simulink model "Robot_diferencial"  (R2017b)
settings: Solver=VariableStepAuto  StartTime=0.0  StopTime=Tsim  MaxStep=1e-2  MinStep=1e-5  RelTol=1e-3
values from neighbouring files (symbols this model uses):
  CI = [0 0 0]    [graf.m]
settings Model: Creator=Raúl  LastModifiedBy=Raúl

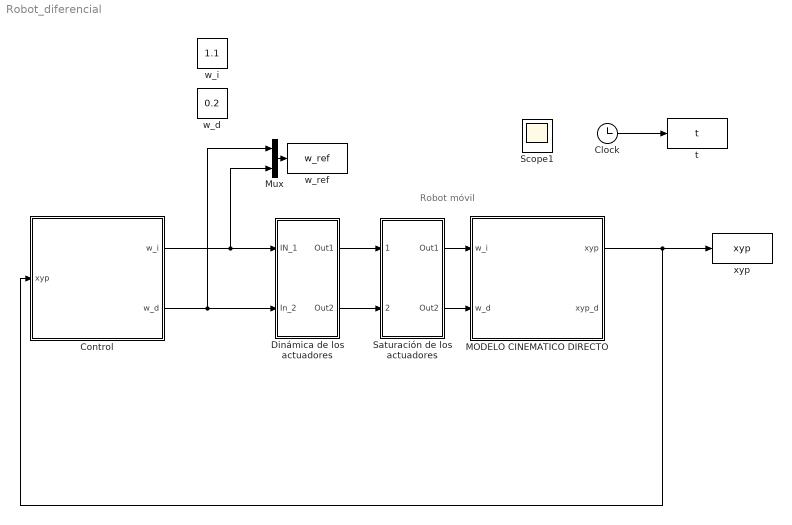
== system Robot_diferencial ==
  note: Robot móvil
  Clock : Clock
  "Control " : Subsystem
  Dinámica de los actuadores : Subsystem
  MODELO CINEMATICO DIRECTO : Subsystem
  Mux : Mux  Inputs=2
  Saturación de los actuadores : Subsystem
  Scope1 : Scope  NumInputPorts=2
  t : ToWorkspace  VariableName=t  SampleTime=-1
  w_d : Constant  Value=0.2
  w_i : Constant  Value=1.1
  w_ref : ToWorkspace  VariableName=w_ref  SampleTime=-1
  xyp : ToWorkspace  VariableName=xyp  SampleTime=-1
  wires:
  MODELO CINEMATICO DIRECTO/1(xyp) -> "Control "/1(xyp), xyp/1
  Clock/1 -> t/1
  Saturación de los actuadores/1(Out1) -> MODELO CINEMATICO DIRECTO/1(w_i)
  Saturación de los actuadores/2(Out2) -> MODELO CINEMATICO DIRECTO/2(w_d)
  Dinámica de los actuadores/1(Out1) -> Saturación de los actuadores/1(w_i_ref)
  Dinámica de los actuadores/2(Out2) -> Saturación de los actuadores/2(w_d_ref)
  "Control "/1(w_i) -> Mux/2, Dinámica de los actuadores/1(IN_1)
  "Control "/2(w_d) -> Mux/1, Dinámica de los actuadores/2(In_2)
  Mux/1 -> w_ref/1

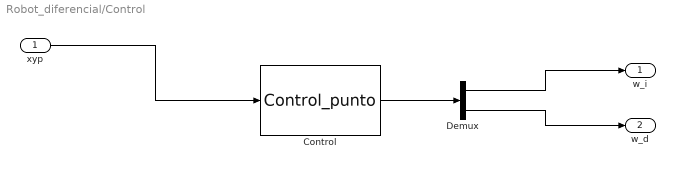
== system Robot_diferencial/Control  ==
  xyp : Inport
  "Control " : MATLABFcn  MATLABFcn=Control_punto
  Demux : Demux  Outputs=2
  w_i : Outport
  w_d : Outport  Port=2
  wires:
  Demux/1 -> w_i/1
  Demux/2 -> w_d/1
  "Control "/1 -> Demux/1
  xyp/1 -> "Control "/1

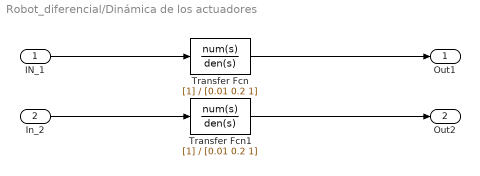
== system Robot_diferencial/Dinámica de los actuadores ==
  IN_1 : Inport
  In_2 : Inport  Port=2
  Transfer Fcn : TransferFcn  Denominator=[0.01 0.2 1]
  Transfer Fcn1 : TransferFcn  Denominator=[0.01 0.2 1]
  Out1 : Outport
  Out2 : Outport  Port=2
  wires:
  Transfer Fcn1/1 -> Out2/1
  In_2/1 -> Transfer Fcn1/1
  Transfer Fcn/1 -> Out1/1
  IN_1/1 -> Transfer Fcn/1

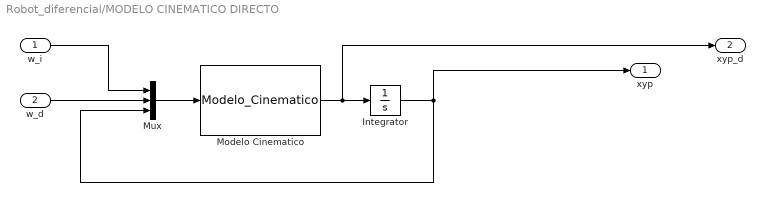
== system Robot_diferencial/MODELO CINEMATICO DIRECTO ==
  w_i : Inport
  w_d : Inport  Port=2
  Integrator : Integrator  InitialCondition=CI
  "Modelo Cinematico " : MATLABFcn  MATLABFcn=Modelo_Cinematico
  Mux : Mux  Inputs=3
  xyp : Outport
  xyp_d : Outport  Port=2
  wires:
  "Modelo Cinematico "/1 -> xyp_d/1, Integrator/1
  w_i/1 -> Mux/1
  Integrator/1 -> xyp/1, Mux/3
  Mux/1 -> "Modelo Cinematico "/1
  w_d/1 -> Mux/2

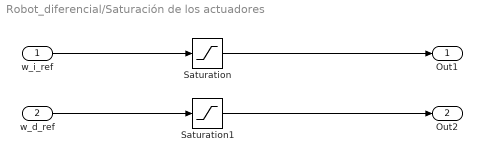
== system Robot_diferencial/Saturación de los actuadores ==
  w_i_ref : Inport
  w_d_ref : Inport  Port=2
  Saturation : Saturate  UpperLimit=2.5  LowerLimit=-2.5
  Saturation1 : Saturate  UpperLimit=2.5  LowerLimit=-2.5
  Out1 : Outport
  Out2 : Outport  Port=2
  wires:
  w_i_ref/1 -> Saturation/1
  Saturation/1 -> Out1/1
  w_d_ref/1 -> Saturation1/1
  Saturation1/1 -> Out2/1
